simulink model "sin_osc"  (R2020a)
settings: Solver=ode14x  StartTime=0.0  StopTime=10.0  FixedStep=0.01  RelTol=1e-3
InitFcn:
  | init_param
values from neighbouring files (symbols this model uses):
  u0 = 0    [init_param.m]
  v0 = 0    [init_param.m]
  w = 4*pi    (= 12.5663706144)    [init_param.m]
settings Model: Creator=QuangDuy  LastModifiedBy=QuangDuy

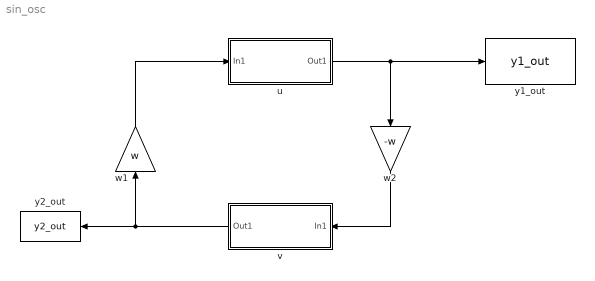
== system sin_osc ==
  u : Subsystem
  v : Subsystem
  w1 : Gain  Gain=w
  w2 : Gain  Gain=-w
  y1_out : ToWorkspace  VariableName=y1_out  SampleTime=-1
  y2_out : ToWorkspace  VariableName=y2_out  SampleTime=-1
  wires:
  w2/1 -> v/1(In1)
  u/1(Out1) -> y1_out/1, w2/1
  w1/1 -> u/1(In1)
  v/1(Out1) -> y2_out/1, w1/1

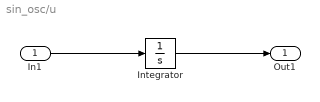
== system sin_osc/u ==
  In1 : Inport
  Integrator : Integrator  InitialCondition=u0
  Out1 : Outport
  wires:
  In1/1 -> Integrator/1
  Integrator/1 -> Out1/1

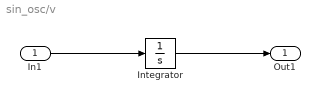
== system sin_osc/v ==
  In1 : Inport
  Integrator : Integrator  InitialCondition=v0
  Out1 : Outport
  wires:
  In1/1 -> Integrator/1
  Integrator/1 -> Out1/1
